simulink model "NeedleValve"  (R2020a)
settings: Solver=VariableStepAuto  StartTime=0.0  StopTime=100  RelTol=1e-3
settings Model: Creator=parthmahendru  LastModifiedBy=parthmahendru

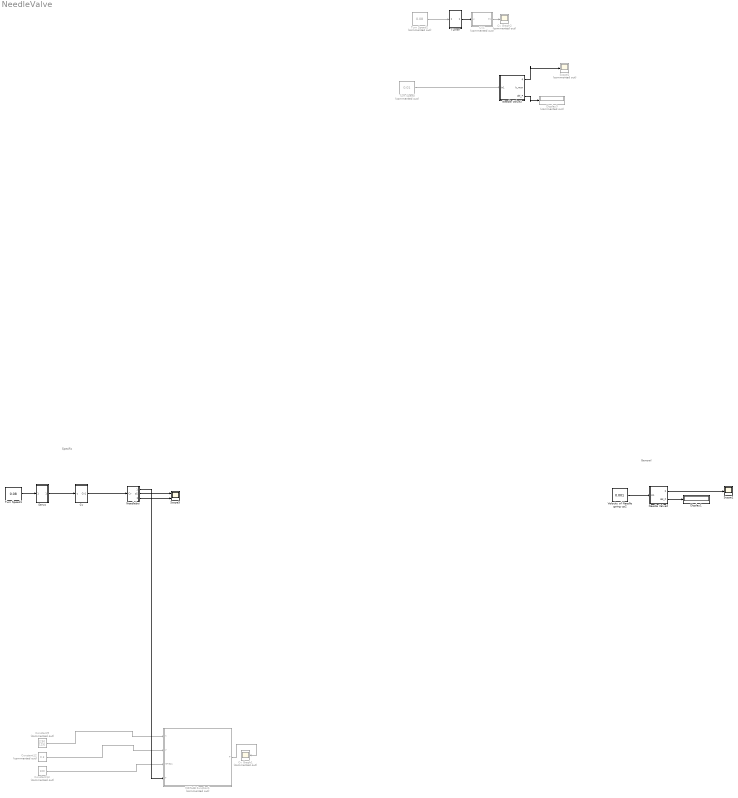
== system NeedleValve ==
  note: Specific
  note: General
  Constant12 : Constant  Commented=on  Value=0.3
  Constant13 : Constant  Commented=on  Value=100
  Constant9 : Constant  Commented=on  Value=[250 125]
  Cv : Subsystem
  Cv Graph1 : Scope  Commented=on
  Cv Graph2 : Scope  Commented=on
  Cv1 : MATLAB Function  Commented=on  TreatAsAtomicUnit=on
  Display1 : Display
  Display3 : Display  Commented=on
  MATLAB Function1 : MATLAB Function  Commented=on  TreatAsAtomicUnit=on
  Needle Valve2 : Subsystem
  Needle Valve3 : Subsystem
  Needleboi : Subsystem
  Scope1 : Scope
  Scope2 : Scope  Commented=on
  Scope5 : Scope  NumInputPorts=2
  Servo : Subsystem
  Turn Speed : Constant  Commented=on  Value=0.01  VectorParams1D=off
  Turn Speed1 : Constant  Value=0.08  VectorParams1D=off
  Turn Speed2 : Constant  Commented=on  Value=0.08  VectorParams1D=off
  Turner : Subsystem
  Velocity of Needle going up2 : Constant  Value=0.001  VectorParams1D=off
  wires:
  Needle Valve2/2(del_P) -> Display1/1
  Needle Valve2/1(q) -> Scope1/1
  Velocity of Needle going up2/1 -> Needle Valve2/1(In1)
  MATLAB Function1/1(P) -> Cv Graph1/1
  Constant9/1 -> MATLAB Function1/1(n)
  Constant12/1 -> MATLAB Function1/2(V)
  Constant13/1 -> MATLAB Function1/3(nPress)
  Cv1/1(Cv) -> Cv Graph2/1
  Turn Speed2/1 -> Turner/1(In1)
  Turner/1(Out1) -> Cv1/1(u)
  Turn Speed1/1 -> Servo/1(In1)
  Servo/1(Out1) -> Cv/1(u)
  Cv/1(Cv1) -> Needleboi/1(Cv)
  Needleboi/1(Out1) -> MATLAB Function1/4(T)
  Needleboi/2(p2) -> Scope5/1
  Needleboi/3(q) -> Scope5/2
  Turn Speed/1 -> Needle Valve3/1(In1)
  Needle Valve3/1(q) -> Scope2/1
  Needle Valve3/3(del_P) -> Display3/1

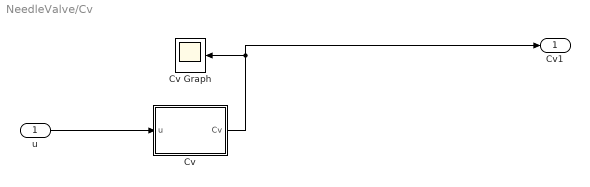
== system NeedleValve/Cv ==
  u : Inport
  Cv : MATLAB Function  TreatAsAtomicUnit=on
  Cv Graph : Scope
  Cv1 : Outport
  wires:
  u/1 -> Cv/1(u)
  Cv/1(Cv) -> Cv1/1, Cv Graph/1

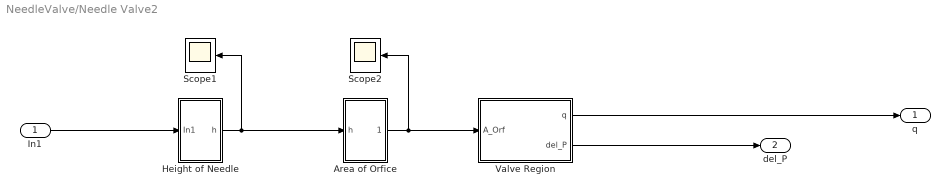
== system NeedleValve/Needle Valve2 ==
  In1 : Inport
  Area of Orfice : Subsystem
  Height of Needle : Subsystem
  Scope1 : Scope
  Scope2 : Scope
  Valve Region : Subsystem
  q : Outport
  del_P : Outport  Port=2
  wires:
  Valve Region/2(del_P) -> del_P/1
  Valve Region/1(q) -> q/1
  Height of Needle/1(h) -> Area of Orfice/1(h), Scope1/1
  In1/1 -> Height of Needle/1(In1)
  Area of Orfice/1(A_Orf) -> Valve Region/1(A_Orf), Scope2/1

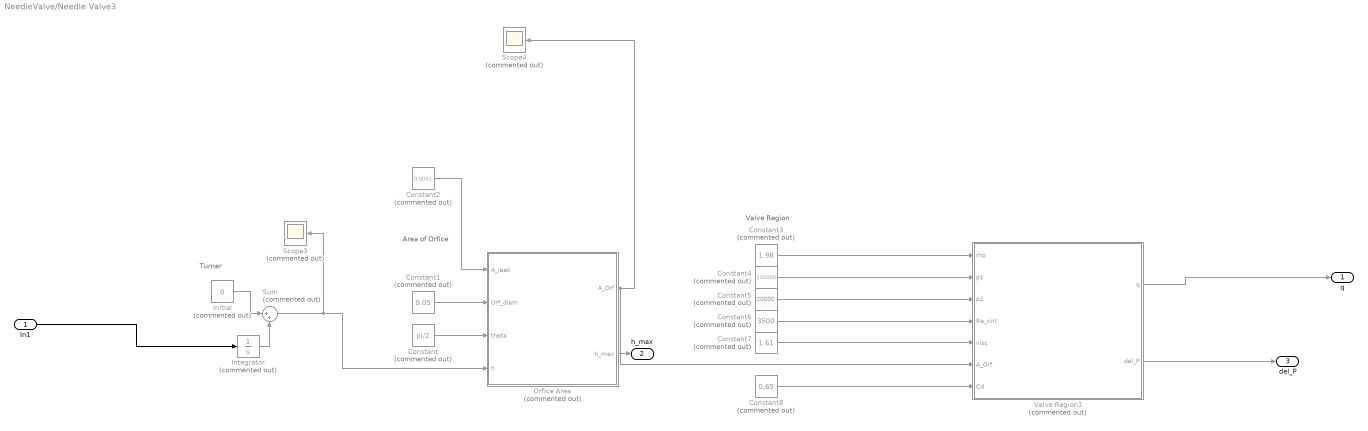
== system NeedleValve/Needle Valve3 ==
  note: Valve Region
  note: Area of Orfice
  note: Turner
  In1 : Inport
  Constant : Constant  Commented=on  Value=pi/2
  Constant1 : Constant  Commented=on  Value=0.05
  Constant2 : Constant  Commented=on  Value=0.0001
  Constant3 : Constant  Commented=on  Value=1.98
  Constant4 : Constant  Commented=on  Value=100000
  Constant5 : Constant  Commented=on  Value=20000
  Constant6 : Constant  Commented=on  Value=3500
  Constant7 : Constant  Commented=on  Value=1.61
  Constant8 : Constant  Commented=on  Value=0.65
  "Initial " : Constant  Commented=on  Value=0
  Integrator : Integrator  Commented=on
  Orfice Area : MATLAB Function  Commented=on  TreatAsAtomicUnit=on
  Scope3 : Scope  Commented=on
  Scope4 : Scope  Commented=on
  Sum : Sum  Commented=on  Inputs=|++
  Valve Region1 : MATLAB Function  Commented=on  TreatAsAtomicUnit=on
  q : Outport
  h_max : Outport  Port=2
  del_P : Outport  Port=3
  wires:
  Valve Region1/2(del_P) -> del_P/1
  Constant1/1 -> Orfice Area/2(Orf_diam)
  "Initial "/1 -> Sum/1
  Constant6/1 -> Valve Region1/4(Re_crit)
  Constant3/1 -> Valve Region1/1(rho)
  Constant5/1 -> Valve Region1/3(p2)
  In1/1 -> Integrator/1
  Valve Region1/1(q) -> q/1
  Sum/1 -> Scope3/1, Orfice Area/4(h)
  Constant2/1 -> Orfice Area/1(A_leak)
  Constant7/1 -> Valve Region1/5(visc)
  Orfice Area/1(A_Orf) -> Valve Region1/6(A_Orf), Scope4/1
  Constant4/1 -> Valve Region1/2(p1)
  Orfice Area/2(h_max) -> h_max/1
  Integrator/1 -> Sum/2
  Constant/1 -> Orfice Area/3(theta)
  Constant8/1 -> Valve Region1/7(Cd)

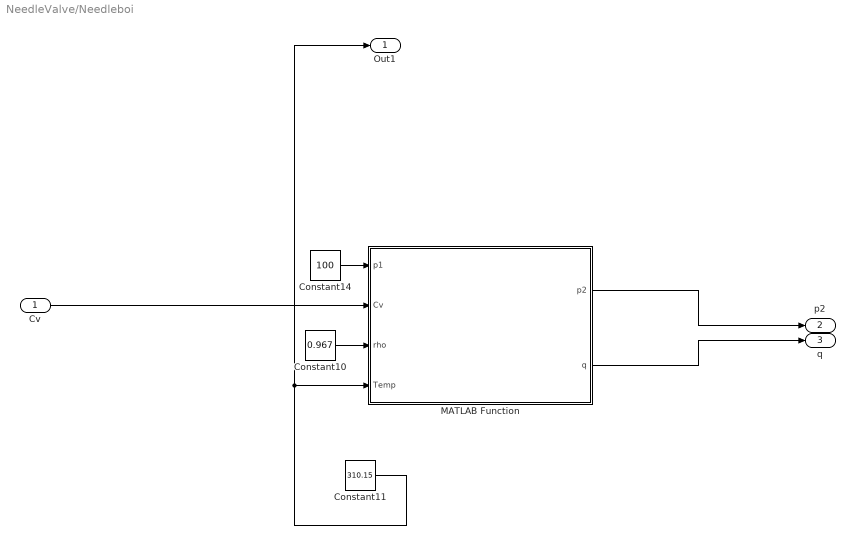
== system NeedleValve/Needleboi ==
  Cv : Inport
  Constant10 : Constant  Value=0.967
  Constant11 : Constant  Value=310.15
  Constant14 : Constant  Value=100
  MATLAB Function : MATLAB Function  TreatAsAtomicUnit=on
  Out1 : Outport
  p2 : Outport  Port=2
  q : Outport  Port=3
  wires:
  Cv/1 -> MATLAB Function/2(Cv)
  Constant10/1 -> MATLAB Function/3(rho)
  Constant14/1 -> MATLAB Function/1(p1)
  MATLAB Function/1(p2) -> p2/1
  MATLAB Function/2(q) -> q/1
  Constant11/1 -> Out1/1, MATLAB Function/4(Temp)

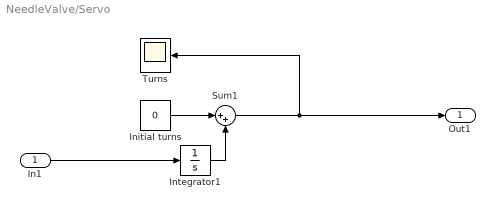
== system NeedleValve/Servo ==
  In1 : Inport
  Initial turns : Constant  Value=0
  Integrator1 : Integrator
  Sum1 : Sum  Inputs=|++
  Turns : Scope
  Out1 : Outport
  wires:
  In1/1 -> Integrator1/1
  Sum1/1 -> Out1/1, Turns/1
  Integrator1/1 -> Sum1/2
  Initial turns/1 -> Sum1/1

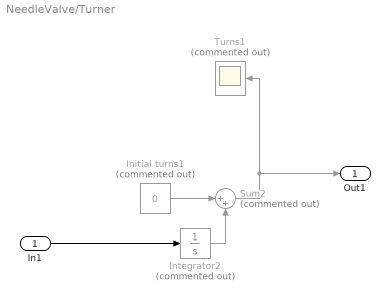
== system NeedleValve/Turner ==
  In1 : Inport
  Initial turns1 : Constant  Commented=on  Value=0
  Integrator2 : Integrator  Commented=on
  Sum2 : Sum  Commented=on  Inputs=|++
  Turns1 : Scope  Commented=on
  Out1 : Outport
  wires:
  Initial turns1/1 -> Sum2/1
  In1/1 -> Integrator2/1
  Integrator2/1 -> Sum2/2
  Sum2/1 -> Out1/1, Turns1/1

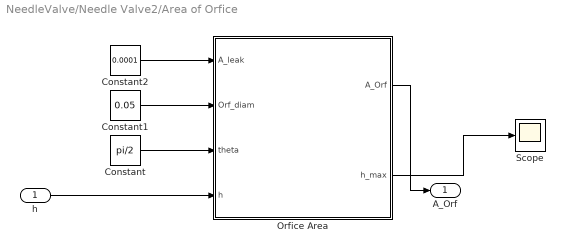
== system NeedleValve/Needle Valve2/Area of Orfice ==
  h : Inport
  Constant : Constant  Value=pi/2
  Constant1 : Constant  Value=0.05
  Constant2 : Constant  Value=0.0001
  Orfice Area : MATLAB Function  TreatAsAtomicUnit=on
  Scope : Scope
  A_Orf : Outport
  wires:
  Constant1/1 -> Orfice Area/2(Orf_diam)
  Constant/1 -> Orfice Area/3(theta)
  h/1 -> Orfice Area/4(h)
  Orfice Area/1(A_Orf) -> A_Orf/1
  Constant2/1 -> Orfice Area/1(A_leak)
  Orfice Area/2(h_max) -> Scope/1

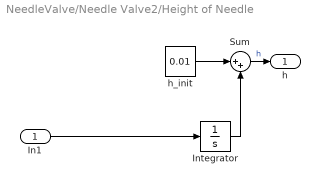
== system NeedleValve/Needle Valve2/Height of Needle ==
  In1 : Inport
  Integrator : Integrator
  Sum : Sum  Inputs=|++
  h_init : Constant  Value=0.01
  h : Outport
  wires:
  In1/1 -> Integrator/1
  Sum/1 -> h/1  "h"
  Integrator/1 -> Sum/2
  h_init/1 -> Sum/1

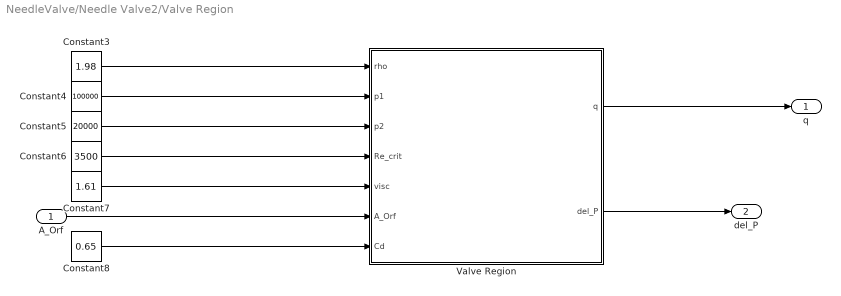
== system NeedleValve/Needle Valve2/Valve Region ==
  A_Orf : Inport
  Constant3 : Constant  Value=1.98
  Constant4 : Constant  Value=100000
  Constant5 : Constant  Value=20000
  Constant6 : Constant  Value=3500
  Constant7 : Constant  Value=1.61
  Constant8 : Constant  Value=0.65
  Valve Region : MATLAB Function  TreatAsAtomicUnit=on
  q : Outport
  del_P : Outport  Port=2
  wires:
  Valve Region/2(del_P) -> del_P/1
  Constant7/1 -> Valve Region/5(visc)
  Constant4/1 -> Valve Region/2(p1)
  Constant8/1 -> Valve Region/7(Cd)
  A_Orf/1 -> Valve Region/6(A_Orf)
  Constant3/1 -> Valve Region/1(rho)
  Constant6/1 -> Valve Region/4(Re_crit)
  Valve Region/1(q) -> q/1
  Constant5/1 -> Valve Region/3(p2)

== matlab function NeedleValve/Cv1 ==
  data: Cv output; u input
function Cv = Cvcalc(u)
if (u<6)
    Cv = u/20;
elseif(u>6&&u<9)
Cv=((1.1169*(u-5.95)^2))/10+0.3;
else
  Cv=0;
    
end

== matlab function NeedleValve/Needle Valve2/Area of Orfice/Orfice Area ==
  data: A_leak input; A_Orf output; Orf_diam input; theta input; h input; h_max output
function [A_Orf, h_max] = OrficeArea(A_leak, Orf_diam, theta, h)
h_max=(Orf_diam*(1-sqrt(1-cos(theta/2))))/sin(theta);

if (h<=0)
    A_Orf= A_leak;
elseif (h>0) && (h<h_max)
    A_Orf=(pi*(Orf_diam-(h*sin(theta/2)*cos(theta/2)))*h*sin(theta/2))+A_leak;
elseif (h>h_max)
    A_Orf=(pi*(Orf_diam)^2/4)+A_leak;
else
    A_Orf=(pi*(Orf_diam)^2/4)+A_leak;
end

%A_Orf=(pi*(Orf_diam)^2/4)+A_leak;

== matlab function NeedleValve/Needle Valve2/Valve Region/Valve Region ==
  data: rho input; q output; p1 input; del_P output; p2 input; Re_crit input; visc input; A_Orf input; Cd input
function[q, del_P] = NeedleValve(rho,p1,p2, Re_crit, visc,A_Orf,Cd)
% theta= angle of tip of needle assuming 90 initially later can be created
% as workspace variable
%h_init = initial height of needle (not 0 prolly for all practical purposes)
%Orf_diam is the diameter of the orfice
%Re_crit is the critical reynolds number
%P_minT is the pressure just before turbulent flow
%q is the mass flow rate
%visc = fluid kinematic viscosity
%del_P is the pressure differential

Dh=sqrt((4*A_Orf)/pi);
del_P=p1-p2;
P_minT=(rho/2)*((Re_crit*visc)/(Cd*Dh))^2;
q=Cd*A_Orf*sqrt(2/rho)*del_P/((((del_P))^2+(P_minT)^2))^0.25;

== matlab function NeedleValve/Needle Valve3/Orfice Area ==
  data: A_leak input; A_Orf output; Orf_diam input; theta input; h input; h_max output
function [A_Orf, h_max] = OrficeArea(A_leak, Orf_diam, theta, h)
h_max=(Orf_diam*(1-sqrt(1-cos(theta/2))))/sin(theta);

if (h<=0)
    A_Orf= A_leak;
elseif (h>0) && (h<h_max)
    A_Orf=(pi*(Orf_diam-(h*sin(theta/2)*cos(theta/2)))*h*sin(theta/2))+A_leak;
elseif (h>h_max)
    A_Orf=(pi*(Orf_diam)^2/4)+A_leak;
else
    A_Orf=(pi*(Orf_diam)^2/4)+A_leak;
end

%A_Orf=(pi*(Orf_diam)^2/4)+A_leak;

== matlab function NeedleValve/Needle Valve3/Valve Region1 ==
  data: rho input; q output; p1 input; del_P output; p2 input; Re_crit input; visc input; A_Orf input; Cd input
function[q, del_P] = NeedleValve(rho,p1,p2, Re_crit, visc,A_Orf,Cd)
% theta= angle of tip of needle assuming 90 initially later can be created
% as workspace variable
%h_init = initial height of needle (not 0 prolly for all practical purposes)
%Orf_diam is the diameter of the orfice
%Re_crit is the critical reynolds number
%q is the mass flow rate
%visc = fluid kinematic viscosity
%del_P is the pressure differential

Dh=sqrt((4*A_Orf)/pi);
del_P=p1-p2;
P_minT=(rho/2)*((Re_crit*visc)/(Cd*Dh))^2;
q=Cd*A_Orf*sqrt(2/rho)*del_P/((((del_P))^2+(P_minT)^2))^0.25;

== matlab function NeedleValve/Cv/Cv ==
  data: Cv output; u input
function Cv = Cvcalc(u)
if (u<6)
    Cv = u/20;
elseif(u>6&&u<9)
Cv=((1.1169*(u-5.95)^2))/10+0.3;
else
  Cv=0;
    
end

== matlab function NeedleValve/Needleboi/MATLAB Function ==
  data: p1 input; p2 output; Cv input; rho input; Temp input; q output
function [p2,q] = Needleboi(p1,Cv,rho,Temp)

del_p=0;

p2=del_p+p1;
del_p=p1-p2;


if (p2>0.5*p1)
    q=1*Cv*p1*(1-(2*del_p)/(3*p1))*sqrt(del_p/(p1*rho*Temp));
    
else
    q=1*Cv*p1*sqrt(1/(rho*Temp));
end

== matlab function NeedleValve/MATLAB Function1 ==
  data: n input; V input; nPress input; P output; T input
function P  = N20Blowdown1_B(n, V, nPress, T)


Q1 = 2.781;    % molar specific volume of liquid N2O [m^3/kmol] coefficients
Q2 = 0.27244;
Q3 = 309.57;
Q4 = 0.2882;

R  = 8314;      %Universal gas constant (J/kmol*K).

% Calculate thermodynamic parameters as functions of temperature:
Vhat_l      = Q2^(1 + (1 - T/Q3)^Q4)/Q1;                    %Molar specific vol. of liq. N2O [m^3/kmol]

%Simplified expression definitions for solution:
P = (nPress + n(2))*R*T/(V - n(1)*Vhat_l);

end
